simulink model "model_bridge_modified"  (R2023a)
settings: Solver=ode4  StartTime=0.0  StopTime=model.tmax  FixedStep=model.dt  RelTol=1e-3
values from neighbouring files (symbols this model uses):
  element : value not decoded    [Elem9_L5_NL4.sldd]
  model : value not decoded    [Elem9_L5_NL4.sldd]
settings Model: DataDictionary=model_bridge.sldd  Creator=glenn  LastModifiedBy=glenn
settings DataIOCC: SaveState=on
settings DebuggingCC: AlgebraicLoopMsg=none

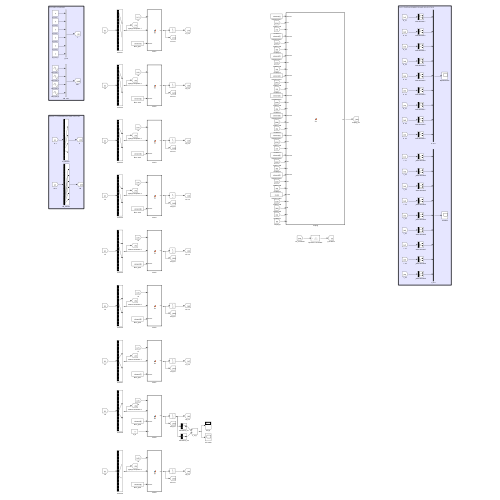
[thumbnail: Simulink's stored preview of the top-level diagram]
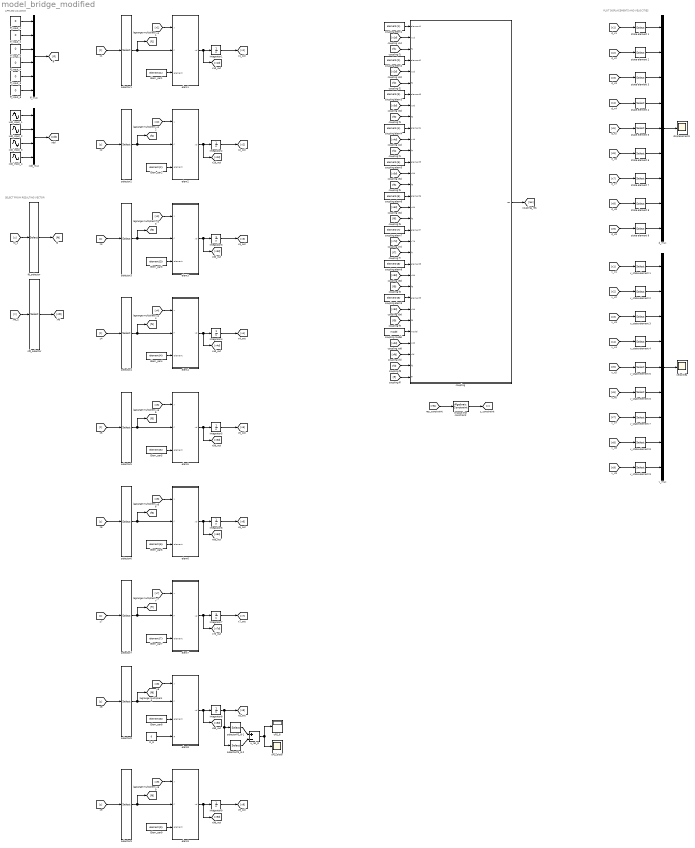
== system model_bridge_modified ==
  note: APPLIED LOADING
  note: SELECT FROM RESULTING VECTOR
  note: PLOT DISPLACEMENTS AND VELOCITIES
  Elem_par1 : Constant  Value=element{1}  OutDataTypeStr=Bus: ePar1
  Elem_par2 : Constant  Value=element{2}  OutDataTypeStr=Bus: ePar2
  Elem_par3 : Constant  Value=element{3}  OutDataTypeStr=Bus: ePar3
  Elem_par4 : Constant  Value=element{4}  OutDataTypeStr=Bus: ePar4
  Elem_par5 : Constant  Value=element{5}  OutDataTypeStr=Bus: ePar5
  Elem_par6 : Constant  Value=element{6}  OutDataTypeStr=Bus: ePar6
  Elem_par7 : Constant  Value=element{7}  OutDataTypeStr=Bus: ePar7
  Elem_par8 : Constant  Value=element{8}  OutDataTypeStr=Bus: ePar8
  Elem_par9 : Constant  Value=element{9}  OutDataTypeStr=Bus: ePar9
  Integrator{1..3,8..9} (5 alike) : Integrator  InitialCondition=zeros(4,1)
  Integrator{4..7} (4 alike) : Integrator  InitialCondition=zeros(5,1)
  R_8 : Constant  Value=0
  coupling : MATLAB Function  TreatAsAtomicUnit=on
  coupling elem1 : Constant  Value=element{1}  OutDataTypeStr=Bus: ePar1
  coupling elem2 : Constant  Value=element{2}  OutDataTypeStr=Bus: ePar2
  coupling elem3 : Constant  Value=element{3}  OutDataTypeStr=Bus: ePar3
  coupling elem4 : Constant  Value=element{4}  OutDataTypeStr=Bus: ePar4
  coupling elem5 : Constant  Value=element{5}  OutDataTypeStr=Bus: ePar5
  coupling elem6 : Constant  Value=element{6}  OutDataTypeStr=Bus: ePar6
  coupling elem7 : Constant  Value=element{7}  OutDataTypeStr=Bus: ePar7
  coupling elem8 : Constant  Value=element{8}  OutDataTypeStr=Bus: ePar8
  coupling elem9 : Constant  Value=element{9}  OutDataTypeStr=Bus: ePar9
  coupling model : Constant  Value=model  OutDataTypeStr=Bus: mPar
  d_mux : Mux  Inputs=9
  displacements : Scope
  elem1 : MATLAB Function  TreatAsAtomicUnit=on
  elem2 : MATLAB Function  TreatAsAtomicUnit=on
  elem3 : MATLAB Function  TreatAsAtomicUnit=on
  elem4 : MATLAB Function  TreatAsAtomicUnit=on
  elem5 : MATLAB Function  TreatAsAtomicUnit=on
  elem6 : MATLAB Function  TreatAsAtomicUnit=on
  elem7 : MATLAB Function  TreatAsAtomicUnit=on
  elem8 : MATLAB Function  TreatAsAtomicUnit=on
  elem9 : MATLAB Function  TreatAsAtomicUnit=on
  fd_selector : Selector  InputPortWidth=28  IndexOptions=Index vector (dialog)  Indices="[19  20  21  22]"  OutputSizes=1
  ff_input_{1..6} (6 alike) : Constant  Value=0
  ff_mux : Mux  Inputs=6
  impose the constraint : AlgebraicConstraint
  selector1 : Selector  InputPortWidth=28  IndexOptions=Index vector (dialog)  Indices="[1  2]"  OutputSizes=1
  selector2 : Selector  InputPortWidth=28  IndexOptions=Index vector (dialog)  Indices="[3  4]"  OutputSizes=1
  selector3 : Selector  InputPortWidth=28  IndexOptions=Index vector (dialog)  Indices="[5  6]"  OutputSizes=1
  selector4 : Selector  InputPortWidth=28  IndexOptions=Index vector (dialog)  Indices="[7  8]"  OutputSizes=1
  selector5 : Selector  InputPortWidth=28  IndexOptions=Index vector (dialog)  Indices="[9  10]"  OutputSizes=1
  selector6 : Selector  InputPortWidth=28  IndexOptions=Index vector (dialog)  Indices="[11  12]"  OutputSizes=1
  selector7 : Selector  InputPortWidth=28  IndexOptions=Index vector (dialog)  Indices="[13  14]"  OutputSizes=1
  selector8 : Selector  InputPortWidth=28  IndexOptions=Index vector (dialog)  Indices="[15  16]"  OutputSizes=1
  selector9 : Selector  InputPortWidth=28  IndexOptions=Index vector (dialog)  Indices="[17  18]"  OutputSizes=1
  selectorPS_8-1 : Selector  InputPortWidth=4  IndexOptions=Index vector (dialog)  Indices=1  OutputSizes=1
  selectorPS_8-2 : Selector  InputPortWidth=4  IndexOptions=Index vector (dialog)  Indices=2  OutputSizes=1
  state element {1..3,8..9} (5 alike) : Selector  InputPortWidth=4  IndexOptions=Index vector (dialog)  Indices=[1 2]  OutputSizes=1
  state element {4..7} (4 alike) : Selector  InputPortWidth=5  IndexOptions=Index vector (dialog)  Indices=[1 2]  OutputSizes=1
  uPS_8 : Display
  uPS_plot8 : Scope
  u_rel_8 : Sum  Inputs=+-
  v_mux : Mux  Inputs=9
  v_state element {1..3,8..9} (5 alike) : Selector  InputPortWidth=4  IndexOptions=Index vector (dialog)  Indices=[3 4]  OutputSizes=1
  v_state element {4..7} (4 alike) : Selector  InputPortWidth=5  IndexOptions=Index vector (dialog)  Indices=[3 4]  OutputSizes=1
  velocities : Scope
  xdd_input_{1..4} (4 alike) : Sin  Amplitude=0.15  Frequency=6.2832  SampleTime=0
  xdd_mux : Mux
  xfd_selector : Selector  InputPortWidth=28  IndexOptions=Index vector (dialog)  Indices="[23  24  25  26  27  28]"  OutputSizes=1
  wires:
  ff_input_1/1 -> ff_mux/1
  ff_input_2/1 -> ff_mux/2
  ff_input_3/1 -> ff_mux/3
  ff_input_4/1 -> ff_mux/4
  ff_input_5/1 -> ff_mux/5
  ff_input_6/1 -> ff_mux/6
  ff_mux/1 -> [ff]
  xdd_input_1/1 -> xdd_mux/1
  xdd_input_2/1 -> xdd_mux/2
  xdd_input_3/1 -> xdd_mux/3
  xdd_input_4/1 -> xdd_mux/4
  xdd_mux/1 -> [xdd]
  [z] -> fd_selector/1
  fd_selector/1 -> [fd]
  [z] -> xfd_selector/1
  xfd_selector/1 -> [xfd]
  [res] -> impose the constraint/1
  impose the constraint/1 -> [z]
  [x1] -> elem1/1(x)
  selector1/1 -> elem1/2(f), [f1]
  [z] -> selector1/1
  Elem_par1/1 -> elem1/3(element)
  elem1/1(xd) -> Integrator1/1, [x1d]
  Integrator1/1 -> [x1]
  coupling elem1/1 -> coupling/1(element1)
  [x1d] -> coupling/2(x1d)
  [f1] -> coupling/3(f1)
  [x2] -> elem2/1(x)
  selector2/1 -> elem2/2(f), [f2]
  [z] -> selector2/1
  Elem_par2/1 -> elem2/3(element)
  elem2/1(xd) -> Integrator2/1, [x2d]
  Integrator2/1 -> [x2]
  coupling elem2/1 -> coupling/4(element2)
  [x2d] -> coupling/5(x2d)
  [f2] -> coupling/6(f2)
  [x3] -> elem3/1(x)
  selector3/1 -> elem3/2(f), [f3]
  [z] -> selector3/1
  Elem_par3/1 -> elem3/3(element)
  elem3/1(xd) -> Integrator3/1, [x3d]
  Integrator3/1 -> [x3]
  coupling elem3/1 -> coupling/7(element3)
  [x3d] -> coupling/8(x3d)
  [f3] -> coupling/9(f3)
  [x4] -> elem4/1(x)
  selector4/1 -> elem4/2(f), [f4]
  [z] -> selector4/1
  Elem_par4/1 -> elem4/3(element)
  elem4/1(xd) -> Integrator4/1, [x4d]
  Integrator4/1 -> [x4]
  coupling elem4/1 -> coupling/10(element4)
  [x4d] -> coupling/11(x4d)
  [f4] -> coupling/12(f4)
  [x5] -> elem5/1(x)
  selector5/1 -> elem5/2(f), [f5]
  [z] -> selector5/1
  Elem_par5/1 -> elem5/3(element)
  elem5/1(xd) -> Integrator5/1, [x5d]
  Integrator5/1 -> [x5]
  coupling elem5/1 -> coupling/13(element5)
  [x5d] -> coupling/14(x5d)
  [f5] -> coupling/15(f5)
  [x6] -> elem6/1(x)
  selector6/1 -> elem6/2(f), [f6]
  [z] -> selector6/1
  Elem_par6/1 -> elem6/3(element)
  elem6/1(xd) -> Integrator6/1, [x6d]
  Integrator6/1 -> [x6]
  coupling elem6/1 -> coupling/16(element6)
  [x6d] -> coupling/17(x6d)
  [f6] -> coupling/18(f6)
  [x7] -> elem7/1(x)
  selector7/1 -> elem7/2(f), [f7]
  [z] -> selector7/1
  Elem_par7/1 -> elem7/3(element)
  elem7/1(xd) -> Integrator7/1, [x7d]
  Integrator7/1 -> [x7]
  coupling elem7/1 -> coupling/19(element7)
  [x7d] -> coupling/20(x7d)
  [f7] -> coupling/21(f7)
  [x8] -> elem8/1(x)
  selector8/1 -> elem8/2(f), [f8]
  [z] -> selector8/1
  Elem_par8/1 -> elem8/3(element)
  elem8/1(xd) -> Integrator8/1, [x8d]
  Integrator8/1 -> selectorPS_8-1/1, selectorPS_8-2/1, [x8]
  coupling elem8/1 -> coupling/22(element8)
  [x8d] -> coupling/23(x8d)
  [f8] -> coupling/24(f8)
  R_8/1 -> elem8/4(R)
  selectorPS_8-1/1 -> u_rel_8/1
  selectorPS_8-2/1 -> u_rel_8/2
  u_rel_8/1 -> uPS_8/1, uPS_plot8/1
  [x9] -> elem9/1(x)
  selector9/1 -> elem9/2(f), [f9]
  [z] -> selector9/1
  Elem_par9/1 -> elem9/3(element)
  elem9/1(xd) -> Integrator9/1, [x9d]
  Integrator9/1 -> [x9]
  coupling elem9/1 -> coupling/25(element9)
  [x9d] -> coupling/26(x9d)
  [f9] -> coupling/27(f9)
  coupling model/1 -> coupling/28(model)
  [xdd] -> coupling/29(xdd)
  [xfd] -> coupling/30(xfd)
  [fd] -> coupling/31(fd)
  [ff] -> coupling/32(ff)
  coupling/1(res) -> [res]
  [x1] -> state element 1/1
  state element 1/1 -> d_mux/1
  [x2] -> state element 2/1
  state element 2/1 -> d_mux/2
  [x3] -> state element 3/1
  state element 3/1 -> d_mux/3
  [x4] -> state element 4/1
  state element 4/1 -> d_mux/4
  [x5] -> state element 5/1
  state element 5/1 -> d_mux/5
  [x6] -> state element 6/1
  state element 6/1 -> d_mux/6
  [x7] -> state element 7/1
  state element 7/1 -> d_mux/7
  [x8] -> state element 8/1
  state element 8/1 -> d_mux/8
  [x9] -> state element 9/1
  state element 9/1 -> d_mux/9
  d_mux/1 -> displacements/1
  [x1] -> v_state element 1/1
  v_state element 1/1 -> v_mux/1
  [x2] -> v_state element 2/1
  v_state element 2/1 -> v_mux/2
  [x3] -> v_state element 3/1
  v_state element 3/1 -> v_mux/3
  [x4] -> v_state element 4/1
  v_state element 4/1 -> v_mux/4
  [x5] -> v_state element 5/1
  v_state element 5/1 -> v_mux/5
  [x6] -> v_state element 6/1
  v_state element 6/1 -> v_mux/6
  [x7] -> v_state element 7/1
  v_state element 7/1 -> v_mux/7
  [x8] -> v_state element 8/1
  v_state element 8/1 -> v_mux/8
  [x9] -> v_state element 9/1
  v_state element 9/1 -> v_mux/9
  v_mux/1 -> velocities/1

== matlab function model_bridge_modified/elem8 ==
  data: x input; xd output; f input; element input; R input
function xd = fcn(x,f,element,R)

k = 7200; % Stiffness of cantilever beam at Aarhus, N/m
r = [k -k; -k k] * x(1:2);
R = [-x(3:4); r];
xd = element.M \ (element.B*f - R);

end

== matlab function model_bridge_modified/elem9 ==
  data: x input; xd output; f input; element input
function xd = fcn(x,f,element)

xd = element.M \ (element.B*f - R_linear(x,element));

end

== matlab function model_bridge_modified/coupling ==
  data: element1 input; res output; x1d input; f1 input; element2 input; x2d input; f2 input; element3 input; x3d input; f3 input; element4 input; x4d input; f4 input; element5 input; x5d input; f5 input; element6 input; x6d input; f6 input; element7 input; x7d input; f7 input; element8 input; x8d input; f8 input; element9 input; x9d input; f9 input; model input; xdd input; xfd input; fd input; ff input
function res = fcn(element1,x1d,f1,element2,x2d,f2,element3,x3d,f3,element4,x4d,f4,element5,x5d,f5,element6,x6d,f6,element7,x7d,f7,element8,x8d,f8,element9,x9d,f9,model,xdd,xfd,fd,ff)

% Equilibrium
epsilon_B = element1.Bbar * f1 + element2.Bbar * f2 + element3.Bbar * f3 + element4.Bbar * f4 + element5.Bbar * f5 + element6.Bbar * f6 + element7.Bbar * f7 + element8.Bbar * f8 + element9.Bbar * f9 + model.Bbar_f * ff + model.Bbar_d * fd;

% Compatibility
epsilon_G = [
element1.G_f * x1d + element1.Gbar_f * xfd ;
element2.G_f * x2d + element2.Gbar_f * xfd ;
element3.G_f * x3d + element3.Gbar_f * xfd ;
[element4.G_f; element4.G_d] * x4d + blkdiag(element4.Gbar_f, element4.Gbar_d) * [xfd; xdd] ;
element5.G_f * x5d + element5.Gbar_f * xfd ;
element6.G_f * x6d + element6.Gbar_f * xfd ;
[element7.G_f; element7.G_d] * x7d + blkdiag(element7.Gbar_f, element7.Gbar_d) * [xfd; xdd] ;
[element8.G_f; element8.G_d] * x8d + blkdiag(element8.Gbar_f, element8.Gbar_d) * [xfd; xdd] ;
[element9.G_f; element9.G_d] * x9d + blkdiag(element9.Gbar_f, element9.Gbar_d) * [xfd; xdd] ;
];

% Residuals
res = [epsilon_B; epsilon_G];

end

== matlab function model_bridge_modified/elem2 ==
  data: x input; xd output; f input; element input
function xd = fcn(x,f,element)

xd = element.M \ (element.B*f - R_linear(x,element));

end

== matlab function model_bridge_modified/elem1 ==
  data: x input; xd output; f input; element input
function xd = fcn(x,f,element)

xd = element.M \ (element.B*f - R_linear(x,element));

end

== matlab function model_bridge_modified/elem3 ==
  data: x input; xd output; f input; element input
function xd = fcn(x,f,element)

xd = element.M \ (element.B*f - R_linear(x,element));

end

== matlab function model_bridge_modified/elem4 ==
  data: x input; xd output; f input; element input
function xd = fcn(x,f,element)

xd = element.M \ (element.B*f - R_mostaghel(x,element));

end

== matlab function model_bridge_modified/elem5 ==
  data: x input; xd output; f input; element input
function xd = fcn(x,f,element)

xd = element.M \ (element.B*f - R_mostaghel(x,element));

end

== matlab function model_bridge_modified/elem6 ==
  data: x input; xd output; f input; element input
function xd = fcn(x,f,element)

xd = element.M \ (element.B*f - R_mostaghel(x,element));

end

== matlab function model_bridge_modified/elem7 ==
  data: x input; xd output; f input; element input
function xd = fcn(x,f,element)

xd = element.M \ (element.B*f - R_mostaghel(x,element));

end
